simulink model "Three_Phase_Full_Wave_Controlled_Bridge_Rectifier"  (R2017b)
settings: Solver=VariableStepAuto  StartTime=0.0  StopTime=1.0  MaxStep=1e-4  RelTol=1e-3
libraries: powerlib x24, powerlib_meascontrol x3
settings Model: Creator=DELL  LastModifiedBy=DELL

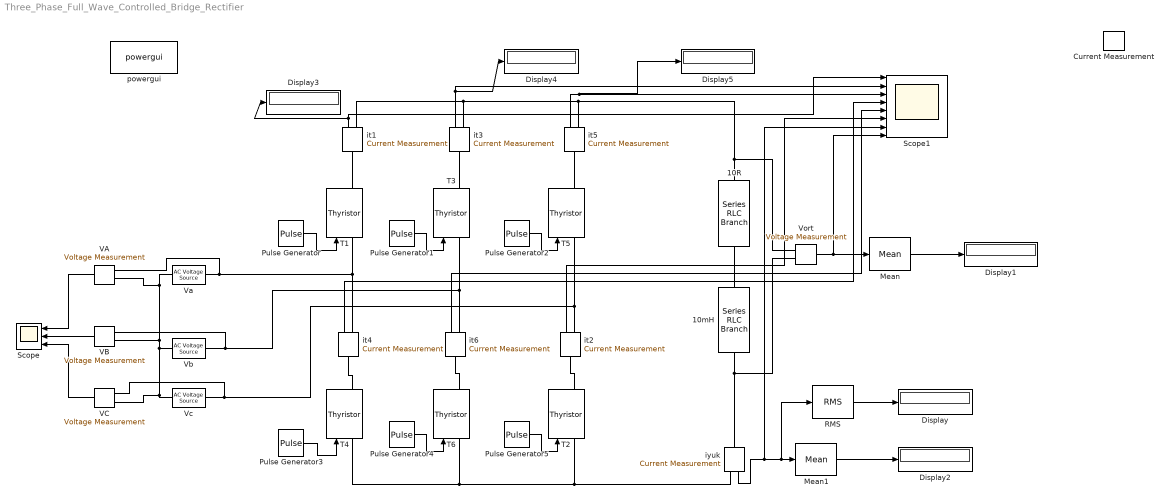
== system Three_Phase_Full_Wave_Controlled_Bridge_Rectifier ==
  10R : powerlib/Elements/Series RLC Branch  LConnTagsString=__new0  RConnTagsString=__new0  BranchType=R  Resistance=10  Inductance=1e-3  SetiL0=off  InitialCurrent=0  Capacitance=1e-6  Setx0=off  InitialVoltage=0  Measurements=None
  10mH : powerlib/Elements/Series RLC Branch  LConnTagsString=__new0  RConnTagsString=__new0  BranchType=L  Resistance=1  Inductance=10e-3  SetiL0=off  InitialCurrent=0  Capacitance=1e-6  Setx0=off  InitialVoltage=0  Measurements=None
  Current Measurement : powerlib/Measurements/Current Measurement  PhasorSimulation=off  OutputType=Complex  PSBequivalent=0
  Display{,1..5} (6 alike) : Display
  Mean : powerlib_meascontrol/Measurements/Mean  Freq=50  Vinit=0  Ts=0
  Mean1 : powerlib_meascontrol/Measurements/Mean  Freq=50  Vinit=0  Ts=0
  Pulse Generator : DiscretePulseGenerator  PulseType=Time based  Period=0.02  PulseWidth=5  PhaseDelay=0.02*120/360
  Pulse Generator1 : DiscretePulseGenerator  PulseType=Time based  Period=0.02  PulseWidth=5  PhaseDelay=0.02*240/360
  Pulse Generator2 : DiscretePulseGenerator  PulseType=Time based  Period=0.02  PulseWidth=5  PhaseDelay=0.02*360/360
  Pulse Generator3 : DiscretePulseGenerator  PulseType=Time based  Period=0.02  PulseWidth=5  PhaseDelay=0.02*300/360
  Pulse Generator4 : DiscretePulseGenerator  PulseType=Time based  Period=0.02  PulseWidth=5  PhaseDelay=0.02*420/360
  Pulse Generator5 : DiscretePulseGenerator  PulseType=Time based  Period=0.02  PulseWidth=5  PhaseDelay=0.02*180/360
  RMS : powerlib_meascontrol/Measurements/RMS  TrueRMS=on  Freq=50  RMSInit=120  Ts=0
  Scope : Scope  NumInputPorts=3
  Scope1 : Scope  NumInputPorts=8
  T{1..6} (6 alike) : powerlib/Power Electronics/Thyristor  Ron=0.001  Lon=0  Vf=0.8  IC=0  Rs=500  Cs=250e-9  Measurements=on
  VA : powerlib/Measurements/Voltage Measurement  PhasorSimulation=off  OutputType=Complex  PSBequivalent=0
  VB : powerlib/Measurements/Voltage Measurement  PhasorSimulation=off  OutputType=Complex  PSBequivalent=0
  VC : powerlib/Measurements/Voltage Measurement  PhasorSimulation=off  OutputType=Complex  PSBequivalent=0
  Va : powerlib/Electrical Sources/AC Voltage Source  Amplitude=311.1269837  Phase=0  Frequency=50  SampleTime=0  Measurements=None  BusType=swing  Pref=10e3  Qref=0  Qmin=-inf  Qmax=+inf
  Vb : powerlib/Electrical Sources/AC Voltage Source  Amplitude=311.1269837  Phase=-120  Frequency=50  SampleTime=0  Measurements=None  BusType=swing  Pref=10e3  Qref=0  Qmin=-inf  Qmax=+inf
  Vc : powerlib/Electrical Sources/AC Voltage Source  Amplitude=311.1269837  Phase=120  Frequency=50  SampleTime=0  Measurements=None  BusType=swing  Pref=10e3  Qref=0  Qmin=-inf  Qmax=+inf
  Vort : powerlib/Measurements/Voltage Measurement  PhasorSimulation=off  OutputType=Complex  PSBequivalent=0
  it{1..6} (6 alike) : powerlib/Measurements/Current Measurement  PhasorSimulation=off  OutputType=Complex  PSBequivalent=0
  iyuk : powerlib/Measurements/Current Measurement  PhasorSimulation=off  OutputType=Complex  PSBequivalent=0
  powergui : powerlib/powergui  Priority=1  SimulationMode=Continuous  SampleTime=50e-6  frequency=60  Iterations=50  frequencyindice=50  Pbase=100e6  ErrMax=1e-4  UnitsV=kV  UnitsW=MW  buscounter=0  FunctionMessages=off  echomessages=off  EnableUseOfTLC=off  CurrentSourceSwitches=off  DisableSnubberDevices=off  DisableRonSwitches=off  DisableVfSwitches=off  DisplayEquations=off  SolverType=Tustin/Backward Euler (TBE)  Interpol=off  ExternalGateDelay=off  methode=off  Ts=100  x0status=blocks  SPID=on  SwTol=0  HookPort=off  RestoreLinks=warning  ResistiveCurrentMeasurement=off  Frange=[0:2:500]  Ylog=off  Xlog=on  ShowGrid=off  save=off  variable=ZData  structure=0  ZoomFFT=off  StartTime=0.0  cycles=1  DisplayStyle=1  fundamental=60  FreqAxis=off  MaxFrequency=1000  frequencyindicesteady=1  RmsSteady=1  display=off
  wires:
  Pulse Generator/1 -> T1/1
  Pulse Generator1/1 -> T3/1
  Pulse Generator2/1 -> T5/1
  Pulse Generator3/1 -> T4/1
  Pulse Generator4/1 -> T6/1
  Pulse Generator5/1 -> T2/1
  VA/1 -> Scope/1
  VB/1 -> Scope/2
  VC/1 -> Scope/3
  Vort/1 -> Scope1/8, Mean/1
  Mean/1 -> Display1/1
  iyuk/1 -> Scope1/7, RMS/1, Mean1/1
  Mean1/1 -> Display2/1
  it1/1 -> Display3/1, Scope1/1
  it3/1 -> Display4/1, Scope1/2
  it5/1 -> Display5/1, Scope1/3
  it4/1 -> Scope1/4
  it6/1 -> Scope1/5
  it2/1 -> Scope1/6
  RMS/1 -> Display/1
  connections:
  Va/RConn1 -- VA/LConn1 -- it4/RConn1 -- T1/LConn1
  T4/RConn1 -- it4/LConn1
  T6/RConn1 -- it6/LConn1
  it6/RConn1 -- VB/LConn1 -- Vb/RConn1 -- T3/LConn1
  it2/LConn1 -- T2/RConn1
  it2/RConn1 -- VC/LConn1 -- Vc/RConn1 -- T5/LConn1
  it5/LConn1 -- T5/RConn1
  it3/LConn1 -- T3/RConn1
  it1/LConn1 -- T1/RConn1
  10mH/RConn1 -- Vort/LConn2 -- iyuk/LConn1
  10mH/LConn1 -- 10R/RConn1
  it5/RConn1 -- Vort/LConn1 -- 10R/LConn1 -- it1/RConn1 -- it3/RConn1
  iyuk/RConn1 -- T4/LConn1 -- T6/LConn1 -- T2/LConn1
  Vb/LConn1 -- VC/LConn2 -- Vc/LConn1 -- VB/LConn2 -- VA/LConn2 -- Va/LConn1
